simulink model "pll_model_2016a"  (R2016a)
settings: Solver=VariableStepAuto  SolverMode=SingleTasking  StartTime=0.0  StopTime=10.0  RelTol=1e-3
values from neighbouring files (symbols this model uses):
  dco_base = round(N*Fref*ts*2^DCO_WL)    [pll_config.m]
  Tref = 1/Fref    (= 1e-07)    [pll_config.m]
libraries: hdlsllib x5
settings Model: Creator=user  LastModifiedBy=honor
settings DataIOCC: ReturnWorkspaceOutputs=on
settings DebuggingCC: SFUnexpectedBacktrackingDiag=error  SFNoUnconditionalDefaultTransitionDiag=error
settings SFSimCC: SimUseLocalCustomCode=on
settings RTWCC: RTWUseLocalCustomCode=on
settings GRTTargetCC: TargetLangStandard=C99 (ISO)  GeneratePreprocessorConditionals=Use local settings
settings ConfigComp: CovMetricSettings=dwe  CovSaveCumulativeToWorkspaceVar=off  CovSaveSingleToWorkspaceVar=off  CovExternalEMLEnable=on

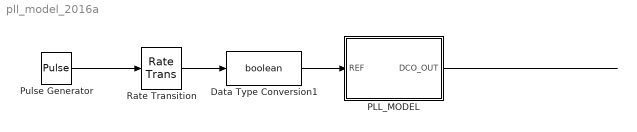
== system pll_model_2016a ==
  Data Type Conversion1 : DataTypeConversion  OutDataTypeStr=boolean  ConvertRealWorld=Stored Integer (SI)
  PLL_MODEL : Subsystem
  Pulse Generator : DiscretePulseGenerator  SampleTime=Tref/2  VectorParams1D=off
  Rate Transition : RateTransition  Integrity=off  Deterministic=off  OutPortSampleTime=ts
  wires:
  Pulse Generator/1 -> Rate Transition/1
  Rate Transition/1 -> Data Type Conversion1/1
  PLL_MODEL/1(DCO_OUT) -> ?
  Data Type Conversion1/1 -> PLL_MODEL/1(REF)

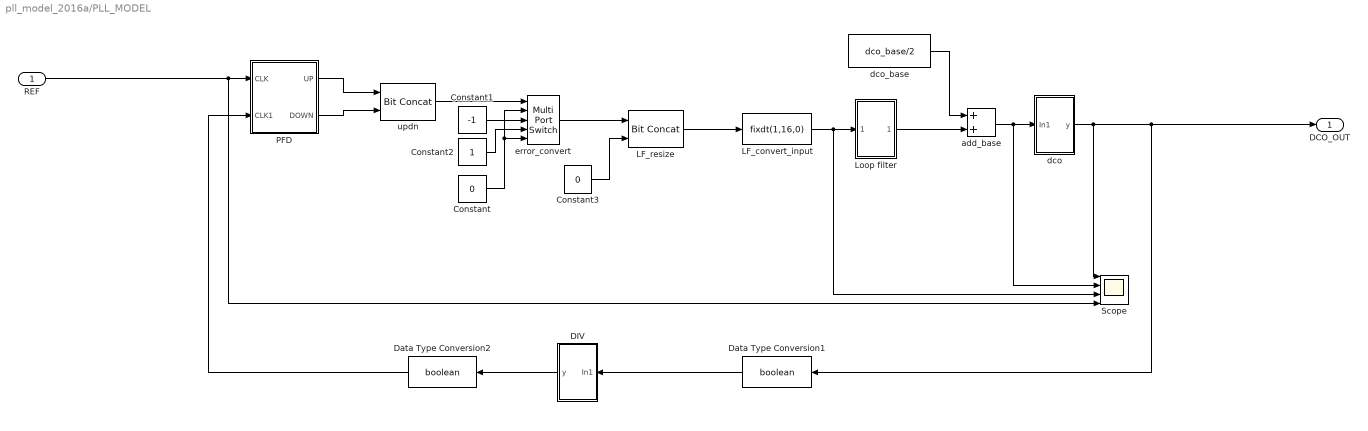
== system pll_model_2016a/PLL_MODEL ==
  REF : Inport
  Constant : Constant  Value=0  OutDataTypeStr=fixdt(1,2,0)
  Constant1 : Constant  Value=-1  OutDataTypeStr=fixdt(1,2,0)
  Constant2 : Constant  OutDataTypeStr=fixdt(1,2,0)
  Constant3 : Constant  Value=0  OutDataTypeStr=fixdt(0,14,0)
  DIV : Subsystem
  Data Type Conversion1 : DataTypeConversion  OutDataTypeStr=boolean  ConvertRealWorld=Stored Integer (SI)
  Data Type Conversion2 : DataTypeConversion  OutDataTypeStr=boolean  ConvertRealWorld=Stored Integer (SI)
  LF_convert_input : DataTypeConversion  OutDataTypeStr=fixdt(1,16,0)  ConvertRealWorld=Stored Integer (SI)
  LF_resize : hdlsllib/HDL Operations/Bit Concat  numInputs=2
  Loop filter : Subsystem
  PFD : Subsystem
  Scope : Scope  NumInputPorts=4
  add_base : Sum  SaturateOnIntegerOverflow=on  OutDataTypeStr=Inherit: Same as first input
  dco : Subsystem
  dco_base : Constant  Value=dco_base/2  OutDataTypeStr=fixdt(1,17,0)
  error_convert : MultiPortSwitch  DataPortOrder=Zero-based contiguous  Inputs=4  zeroidx=on
  updn : hdlsllib/HDL Operations/Bit Concat  numInputs=2
  DCO_OUT : Outport
  wires:
  PFD/2(DOWN) -> updn/2
  LF_convert_input/1 -> Scope/3, Loop filter/1(In1)
  LF_resize/1 -> LF_convert_input/1
  Constant/1 -> error_convert/5, error_convert/2
  Constant2/1 -> error_convert/4
  Constant1/1 -> error_convert/3
  Loop filter/1(Out1) -> add_base/2
  PFD/1(UP) -> updn/1
  error_convert/1 -> LF_resize/1
  dco_base/1 -> add_base/1
  dco/1(y) -> Scope/1, DCO_OUT/1, Data Type Conversion1/1
  REF/1 -> Scope/4, PFD/1(CLK)
  updn/1 -> error_convert/1
  add_base/1 -> Scope/2, dco/1(In1)
  Constant3/1 -> LF_resize/2
  Data Type Conversion1/1 -> DIV/1(In1)
  DIV/1(y) -> Data Type Conversion2/1
  Data Type Conversion2/1 -> PFD/2(CLK1)

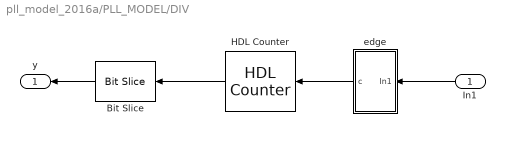
== system pll_model_2016a/PLL_MODEL/DIV ==
  In1 : Inport
  Bit Slice : hdlsllib/HDL Operations/Bit Slice  lidx=3  ridx=3
  HDL Counter : hdlsllib/HDL Operations/HDL Counter  CountType=Free running  CountInit=0  CountStep=1  CountMax=25  CountFromType=Initial value  CountFrom=0  CountResetPort=off  CountLoadPort=off  CountEnbPort=on  CountDirPort=off  CountDataType=Unsigned  CountWordLen=5  CountFracLen=0  CountSampTime=1
  edge : Subsystem
  y : Outport
  wires:
  HDL Counter/1 -> Bit Slice/1
  In1/1 -> edge/1(In1)
  edge/1(c) -> HDL Counter/1
  Bit Slice/1 -> y/1

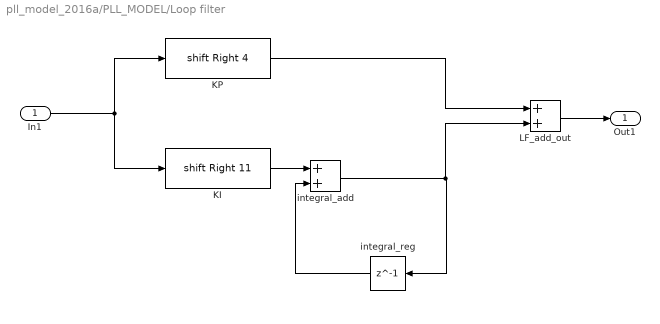
== system pll_model_2016a/PLL_MODEL/Loop filter ==
  In1 : Inport
  KI : ArithShift  BitShiftNumber=11  BitShiftDirection=Right
  KP : ArithShift  BitShiftNumber=4  BitShiftDirection=Right
  LF_add_out : Sum  OutDataTypeStr=fixdt(1,17,0)
  integral_add : Sum  SaturateOnIntegerOverflow=on
  integral_reg : Delay  DelayLength=1  InitialCondition=0
  Out1 : Outport
  wires:
  In1/1 -> KP/1, KI/1
  integral_add/1 -> LF_add_out/2, integral_reg/1
  KI/1 -> integral_add/1
  integral_reg/1 -> integral_add/2
  KP/1 -> LF_add_out/1
  LF_add_out/1 -> Out1/1

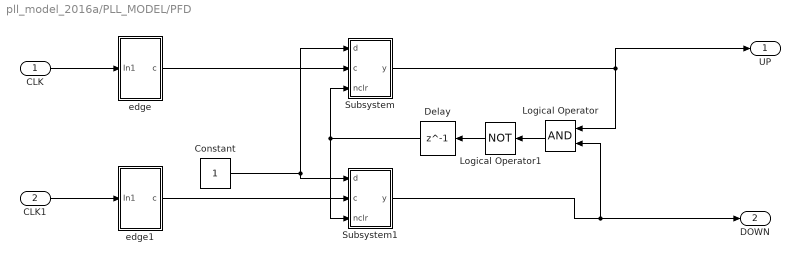
== system pll_model_2016a/PLL_MODEL/PFD ==
  CLK : Inport
  CLK1 : Inport  Port=2
  Constant : Constant  OutDataTypeStr=boolean
  Delay : Delay  DelayLength=1  InitialCondition=0
  Logical Operator : Logic  AllPortsSameDT=off  OutDataTypeStr=boolean
  Logical Operator1 : Logic  Operator=NOT  AllPortsSameDT=off  OutDataTypeStr=boolean
  Subsystem : Subsystem
  Subsystem1 : Subsystem
  edge : Subsystem
  edge1 : Subsystem
  UP : Outport
  DOWN : Outport  Port=2
  wires:
  Logical Operator/1 -> Logical Operator1/1
  Delay/1 -> Subsystem1/3(nclr), Subsystem/3(nclr)
  Constant/1 -> Subsystem1/1(d), Subsystem/1(d)
  Logical Operator1/1 -> Delay/1
  CLK1/1 -> edge1/1(In1)
  CLK/1 -> edge/1(In1)
  Subsystem/1(y) -> UP/1, Logical Operator/1
  edge/1(c) -> Subsystem/2(c)
  edge1/1(c) -> Subsystem1/2(c)
  Subsystem1/1(y) -> Logical Operator/2, DOWN/1

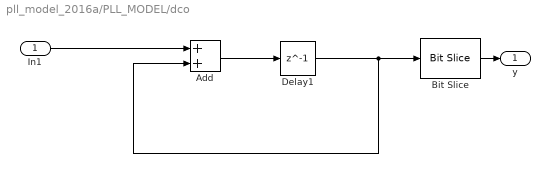
== system pll_model_2016a/PLL_MODEL/dco ==
  In1 : Inport
  Add : Sum  OutDataTypeStr=Inherit: Same as first input
  Bit Slice : hdlsllib/HDL Operations/Bit Slice  lidx=16  ridx=16
  Delay1 : Delay  DelayLength=1  InitialCondition=0
  y : Outport
  wires:
  Add/1 -> Delay1/1
  Delay1/1 -> Add/2, Bit Slice/1
  In1/1 -> Add/1
  Bit Slice/1 -> y/1

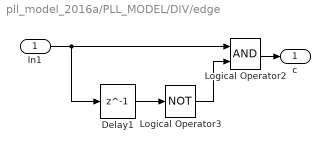
== system pll_model_2016a/PLL_MODEL/DIV/edge ==
  In1 : Inport
  Delay1 : Delay  DelayLength=1  InitialCondition=0
  Logical Operator2 : Logic  AllPortsSameDT=off  OutDataTypeStr=boolean
  Logical Operator3 : Logic  Operator=NOT  AllPortsSameDT=off  OutDataTypeStr=boolean
  c : Outport
  wires:
  Delay1/1 -> Logical Operator3/1
  Logical Operator3/1 -> Logical Operator2/2
  In1/1 -> Delay1/1, Logical Operator2/1
  Logical Operator2/1 -> c/1

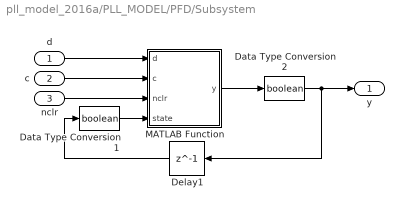
== system pll_model_2016a/PLL_MODEL/PFD/Subsystem ==
  d : Inport
  c : Inport  Port=2
  nclr : Inport  Port=3
  Data Type Conversion1 : DataTypeConversion  OutDataTypeStr=boolean  ConvertRealWorld=Stored Integer (SI)
  Data Type Conversion2 : DataTypeConversion  OutDataTypeStr=boolean  ConvertRealWorld=Stored Integer (SI)
  Delay1 : Delay  DelayLength=1  InitialCondition=0
  MATLAB Function : MATLAB Function  TreatAsAtomicUnit=on
  y : Outport
  wires:
  MATLAB Function/1(y) -> Data Type Conversion2/1
  d/1 -> MATLAB Function/1(d)
  c/1 -> MATLAB Function/2(c)
  nclr/1 -> MATLAB Function/3(nclr)
  Delay1/1 -> Data Type Conversion1/1
  Data Type Conversion1/1 -> MATLAB Function/4(state)
  Data Type Conversion2/1 -> Delay1/1, y/1

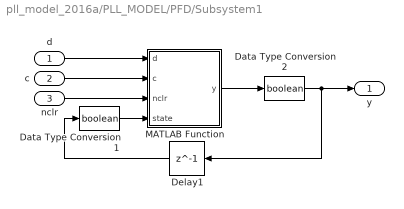
== system pll_model_2016a/PLL_MODEL/PFD/Subsystem1 ==
  d : Inport
  c : Inport  Port=2
  nclr : Inport  Port=3
  Data Type Conversion1 : DataTypeConversion  OutDataTypeStr=boolean  ConvertRealWorld=Stored Integer (SI)
  Data Type Conversion2 : DataTypeConversion  OutDataTypeStr=boolean  ConvertRealWorld=Stored Integer (SI)
  Delay1 : Delay  DelayLength=1  InitialCondition=0
  MATLAB Function : MATLAB Function  TreatAsAtomicUnit=on
  y : Outport
  wires:
  Data Type Conversion2/1 -> y/1, Delay1/1
  Data Type Conversion1/1 -> MATLAB Function/4(state)
  Delay1/1 -> Data Type Conversion1/1
  nclr/1 -> MATLAB Function/3(nclr)
  c/1 -> MATLAB Function/2(c)
  d/1 -> MATLAB Function/1(d)
  MATLAB Function/1(y) -> Data Type Conversion2/1

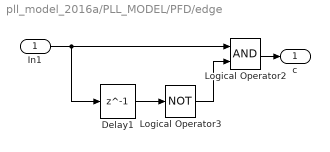
== system pll_model_2016a/PLL_MODEL/PFD/edge ==
  In1 : Inport
  Delay1 : Delay  DelayLength=1  InitialCondition=0
  Logical Operator2 : Logic  AllPortsSameDT=off  OutDataTypeStr=boolean
  Logical Operator3 : Logic  Operator=NOT  AllPortsSameDT=off  OutDataTypeStr=boolean
  c : Outport
  wires:
  Delay1/1 -> Logical Operator3/1
  Logical Operator3/1 -> Logical Operator2/2
  In1/1 -> Delay1/1, Logical Operator2/1
  Logical Operator2/1 -> c/1

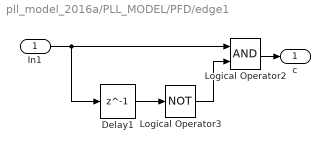
== system pll_model_2016a/PLL_MODEL/PFD/edge1 ==
  In1 : Inport
  Delay1 : Delay  DelayLength=1  InitialCondition=0
  Logical Operator2 : Logic  AllPortsSameDT=off  OutDataTypeStr=boolean
  Logical Operator3 : Logic  Operator=NOT  AllPortsSameDT=off  OutDataTypeStr=boolean
  c : Outport
  wires:
  Logical Operator2/1 -> c/1
  In1/1 -> Logical Operator2/1, Delay1/1
  Logical Operator3/1 -> Logical Operator2/2
  Delay1/1 -> Logical Operator3/1

== matlab function pll_model_2016a/PLL_MODEL/PFD/Subsystem1/MATLAB Function ==
  data: d input; y output; c input; nclr input; state input
function y = fcn(d, c, nclr, state)

if (nclr == 0)
    y = false;
elseif (c == 1)
    y = true;
else
    y = state;
end

== matlab function pll_model_2016a/PLL_MODEL/PFD/Subsystem/MATLAB Function ==
  data: d input; y output; c input; nclr input; state input
function y = fcn(d, c, nclr, state)

if (nclr == 0)
    y = false;
elseif (c == 1)
    y = true;
else
    y = state;
end
